simulink model "qNetwork2"  (R2016a)
settings: Solver=ode45  StartTime=0.0  StopTime=2500  RelTol=1e-3
libraries: commrandsrc3 x1
settings Model: Creator=eiseles  LastModifiedBy=demo
settings DataIOCC: LimitDataPoints=on  SaveFormat=Array
settings DebuggingCC: UnderspecifiedInitializationDetection=Classic  MergeDetectMultiDrivingBlocksExec=none  SolverPrmCheckMsg=warning  StateNameClashWarn=warning
settings HardwareCC: ProdBitPerPointer=32  ProdLargestAtomicFloat=None  ProdIntDivRoundTo=Undefined  ProdEndianess=Unspecified  ProdWordSize=32  ProdHWDeviceType=32-bit Generic
settings ModelReferenceCC: PropagateSignalLabelsOutOfModel=off
settings ConfigComp: CovModelRefEnable=Off
settings SimEventsCC: propMaxDesBlkSimulEvents=2000

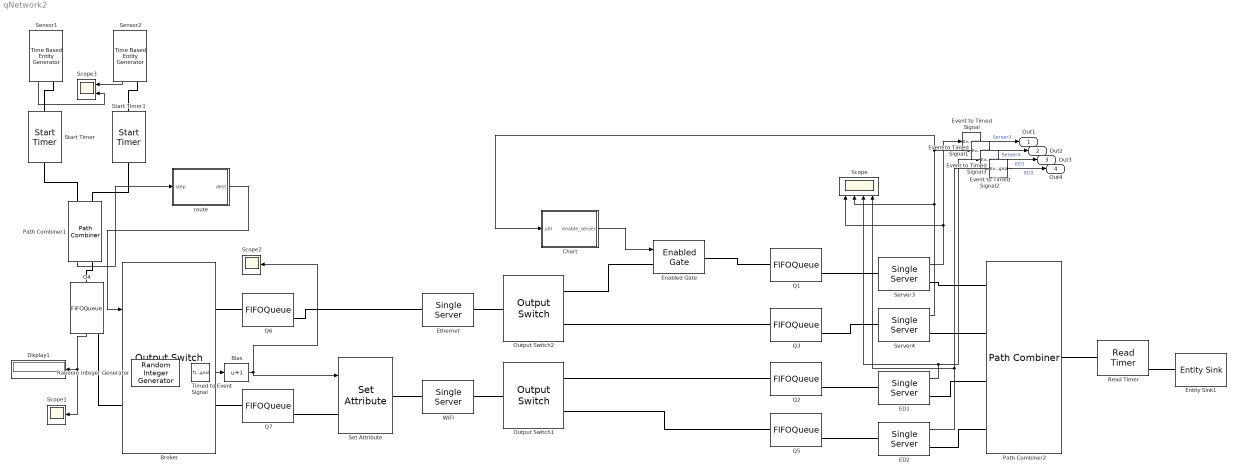
== system qNetwork2 ==
  Bias : Bias  Bias=1
  Broker : OutputSwitch  NumberOutputPorts=2  SwitchingCriterion=From signal port p
  Chart : Stateflow chart  TreatAsAtomicUnit=on
  Display1 : Display
  ED1 : SingleServer  ServiceTime=10  StatUtilization=on
      settings: OutputPortMap=o5
  ED2 : SingleServer  ServiceTime=20  StatUtilization=on
      settings: OutputPortMap=o5
  Enabled Gate : EnabledGate
  Entity Sink1 : EntitySink
  Ethernet : SingleServer  ServiceTime=10
  Event to Timed Signal{,1..3} (4 alike) : EventToTimedSignal
  Output Switch1 : OutputSwitch  NumberOutputPorts=2  SwitchingCriterion=From attribute  AttributeName=dest
  Output Switch2 : OutputSwitch  NumberOutputPorts=2  SwitchingCriterion=Equiprobable
  Path Combiner1 : PathCombiner  NumberInputPorts=2  StatNumberDeparted=on
  Path Combiner2 : PathCombiner  NumberInputPorts=4
  Q{1..3,5..7} (6 alike) : FIFOQueue  Capacity=inf  StatNumberInBlock=on
      settings: OutputPortMap=o1
  Q4 : FIFOQueue  Capacity=inf  StatNumberDeparted=on  StatNumberInBlock=on
      settings: OutputPortMap=o0,o1
  Random Integer Generator : commrandsrc3/Random Integer Generator  SetSize=2  SeedSource=Auto  Seed=0  SampleTime=1  SamplesPerFrame=1  OutputDataType=uint8  SimulateUsing=Interpreted execution
  Read Timer : ReadTimer  TimerModeOption=Ignore  StatTimerNumberDeparted=on  StatAverageTimeElapsed=on
      settings: OutputPortMap=o1,o3
  Scope : Scope  NumInputPorts=4
  Scope1 : Scope
  Scope2 : Scope
  Scope3 : Scope  NumInputPorts=2
  Sensor1 : TimeBasedEntityGenerator  Period=20  GenerateEntityAtSimulationStart=off  StatNumberDeparted=on
  Sensor2 : TimeBasedEntityGenerator  Period=15  GenerateEntityAtSimulationStart=off  StatNumberDeparted=on
  Server3 : SingleServer  ServiceTime=20  StatUtilization=on
      settings: OutputPortMap=o5
  Server4 : SingleServer  ServiceTime=20  StatUtilization=on
      settings: OutputPortMap=o5
  Set Attribute : SetAttribute  AttributeName=dest  AttributeFrom=Signal port  EvaluatedAttributeValue={ []}
  Start Timer : StartTimer
  Start Timer1 : StartTimer  TimerTag=T2
  Timed to Event Signal : TimedToEventSignal
  WiFI : SingleServer  ServiceTime=10
  route : Stateflow chart  TreatAsAtomicUnit=on
  Out1 : Outport
  Out2 : Outport  Port=2
  Out3 : Outport  Port=3
  Out4 : Outport  Port=4
  wires:
  Server4/1 -> Event to Timed Signal1/1, Chart/1(util), Scope/2
  Chart/1(enable_server) -> Enabled Gate/1
  ED1/1 -> Scope/3, Event to Timed Signal2/1
  ED2/1 -> Event to Timed Signal3/1, Scope/4
  Q4/2 -> Scope1/1, Display1/1
  Bias/1 -> Set Attribute/1, Scope2/1
  Random Integer Generator/1 -> Timed to Event Signal/1
  Timed to Event Signal/1 -> Bias/1
  Sensor2/1 -> Scope3/1
  Sensor1/1 -> Scope3/2
  route/1(dest) -> Broker/1
  Path Combiner1/1 -> route/1(step)
  Server3/1 -> Event to Timed Signal/1, Scope/1
  Event to Timed Signal/1 -> Out1/1  "Server3"
  Event to Timed Signal1/1 -> Out2/1  "Server4"
  Event to Timed Signal2/1 -> Out3/1  "ED1"
  Event to Timed Signal3/1 -> Out4/1  "ED2"
  connections:
  Sensor2/RConn1 -- Start Timer1/LConn1
  Sensor1/RConn1 -- Start Timer/LConn1
  Q3/RConn1 -- Server4/LConn1
  Start Timer/RConn1 -- Path Combiner1/LConn1
  Start Timer1/RConn1 -- Path Combiner1/LConn2
  Q4/LConn1 -- Path Combiner1/RConn1
  Q4/RConn1 -- Broker/LConn1
  Server3/RConn1 -- Path Combiner2/LConn1
  Server4/RConn1 -- Path Combiner2/LConn2
  Read Timer/LConn1 -- Path Combiner2/RConn1
  Entity Sink1/LConn1 -- Read Timer/RConn1
  ED1/RConn1 -- Path Combiner2/LConn3
  ED2/RConn1 -- Path Combiner2/LConn4
  Output Switch1/LConn1 -- WiFI/RConn1
  Q2/RConn1 -- ED1/LConn1
  ED2/LConn1 -- Q5/RConn1
  Broker/RConn2 -- Q7/LConn1
  Output Switch2/LConn1 -- Ethernet/RConn1
  Q6/RConn1 -- Ethernet/LConn1
  Set Attribute/RConn1 -- WiFI/LConn1
  Q1/RConn1 -- Server3/LConn1
  Output Switch1/RConn1 -- Q2/LConn1
  Q5/LConn1 -- Output Switch1/RConn2
  Q6/LConn1 -- Broker/RConn1
  Q7/RConn1 -- Set Attribute/LConn1
  Output Switch2/RConn2 -- Q3/LConn1
  Output Switch2/RConn1 -- Enabled Gate/LConn1
  Enabled Gate/RConn1 -- Q1/LConn1

== stateflow chart qNetwork2/route ==
  state Route1
    en: x = 1;
    en: dest = x;
    du: dest = 1;
    du: x = x+1;
  state Route2
    en: x = 1
    en: dest = x
    du: dest = 2
    du: x = x+1
  (default) -> Route1
  Route2 -> Route1 : [x>10]
  Route1 -> Route2 : [x>3]
  data: dest output; x local; step input

== stateflow chart qNetwork2/Chart ==
  state OneServer
  state TwoServers
    en: send(enable_server)
  (default) -> OneServer
  OneServer -> TwoServers : [util>.7]
  TwoServers -> OneServer : [util<.4]
  data: util input
  events: enable_server output EITHER_EDGE_EVENT
